simulink model "Statechart_Capsuleuse"  (R2023a)
settings: Solver=FixedStepAuto  StartTime=0.0  StopTime=inf  RelTol=1e-3  EnableMultiTasking=on
libraries: arduinolib x29, simulink x6
settings Model: SimulationMode=external  ExtModeTrigDuration=2  Creator=Renaud  LastModifiedBy=renaud.costadoat
settings SolverCC: AlgebraicLoopSolver=TrustRegion
settings OptimizationCC: EnhancedBackFolding=on  PassReuseOutputArgsAs=Individual arguments  ZeroExternalMemoryAtStartup=off  ZeroInternalMemoryAtStartup=off  MaxStackSize=64  OptimizeBlockOrder=speed  DifferentSizesBufferReuse=on  OptimizationCustomize=off  EfficientTunableParamExpr=on
settings DebuggingCC: ParameterTunabilityLossMsg=error  UnconnectedInputMsg=warning  UnconnectedOutputMsg=warning  UnconnectedLineMsg=warning
settings HardwareCC: ProdBitPerInt=16  ProdBitPerPointer=16  ProdBitPerSizeT=16  ProdBitPerPtrDiffT=16  ProdLargestAtomicFloat=None  ProdWordSize=8  ProdHWDeviceType=Atmel->AVR
settings ModelReferenceCC: EnableRefExpFcnMdlSchedulingChecks=on
settings SFSimCC: MATLABDynamicMemAlloc=off
settings RTWCC: Description=Embedded Coder  SystemTargetFile=ert.tlc  HardwareBoard=Arduino Mega 2560  TemplateMakefile=ert_default_tmf  GenerateReport=on  Toolchain=Arduino AVR  BuildConfiguration=Faster Runs  IncludeHyperlinkInReport=on  LaunchReport=on  GenerateTraceInfo=on  GenerateTraceReport=on  GenerateTraceReportSl=on  GenerateTraceReportSf=on  GenerateTraceReportEml=on
settings CodeAppCC: ForceParamTrailComments=on  IgnoreCustomStorageClasses=off  OperatorAnnotations=on  SimulinkDataObjDesc=on  SFDataObjDesc=on  InsertBlockDesc=on
settings ERTTargetCC: SupportContinuousTime=on  SupportVariableSizeSignals=on  ExtMode=on  ExtModeTransport=3  ExtModeStaticAlloc=on  ExtModeStaticAllocSize=2048  ExtModeMexFile=ext_xcp  ExtModeMexArgs=0 4 921600  ExtModeIntrfLevel=Level2 - Open

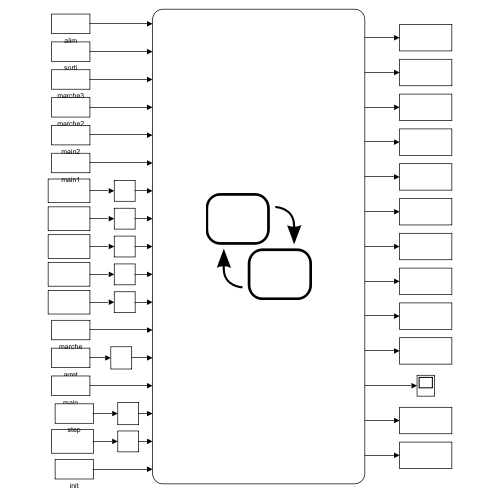
[thumbnail: Simulink's stored preview of the top-level diagram]
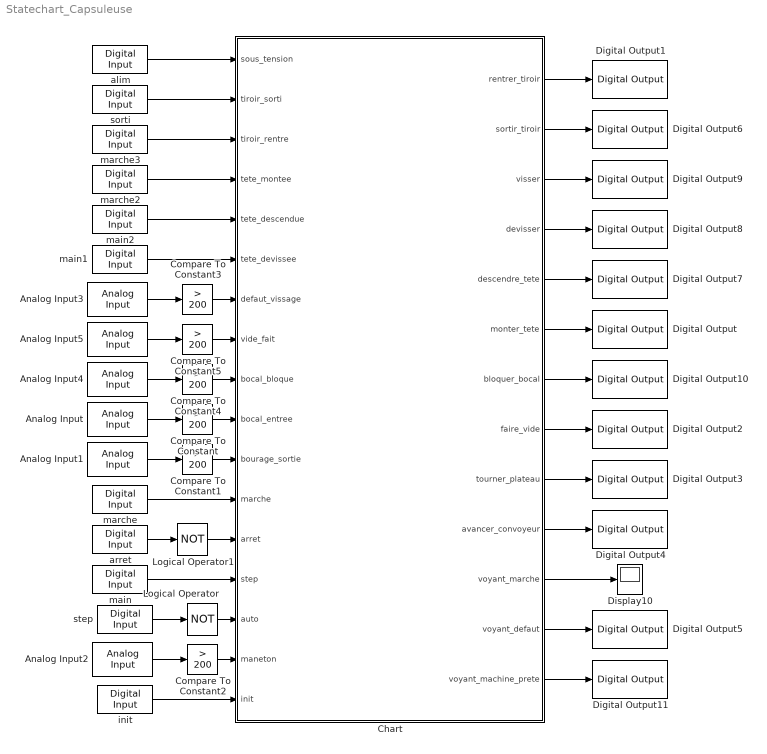
== system Statechart_Capsuleuse ==
  Analog Input : arduinolib/Analog Input  pinNumber=4  ReadResultsOnly=off  ConversionTriggerSource=Software  ExternalTriggerType=uint32( 0 )  OutputDataType=uint16  EnableConversionCompleteNotify=off  EnableOuputStatus=off  SampleTime=-1  blockPlatform=arduino
  Analog Input1 : arduinolib/Analog Input  pinNumber=5  ReadResultsOnly=off  ConversionTriggerSource=Software  ExternalTriggerType=uint32( 0 )  OutputDataType=uint16  EnableConversionCompleteNotify=off  EnableOuputStatus=off  SampleTime=-1  blockPlatform=arduino
  Analog Input2 : arduinolib/Analog Input  pinNumber=3  ReadResultsOnly=off  ConversionTriggerSource=Software  ExternalTriggerType=uint32( 0 )  OutputDataType=uint16  EnableConversionCompleteNotify=off  EnableOuputStatus=off  SampleTime=-1  blockPlatform=arduino
  Analog Input3 : arduinolib/Analog Input  pinNumber=6  ReadResultsOnly=off  ConversionTriggerSource=Software  ExternalTriggerType=uint32( 0 )  OutputDataType=uint16  EnableConversionCompleteNotify=off  EnableOuputStatus=off  SampleTime=-1  blockPlatform=arduino
  Analog Input4 : arduinolib/Analog Input  pinNumber=2  ReadResultsOnly=off  ConversionTriggerSource=Software  ExternalTriggerType=uint32( 0 )  OutputDataType=uint16  EnableConversionCompleteNotify=off  EnableOuputStatus=off  SampleTime=-1  blockPlatform=arduino
  Analog Input5 : arduinolib/Analog Input  pinNumber=1  ReadResultsOnly=off  ConversionTriggerSource=Software  ExternalTriggerType=uint32( 0 )  OutputDataType=uint16  EnableConversionCompleteNotify=off  EnableOuputStatus=off  SampleTime=-1  blockPlatform=arduino
  Chart : Stateflow chart  TreatAsAtomicUnit=on
  Compare To Constant{,1..5} (6 alike) : simulink/Logic and Bit Operations/Compare To Constant  relop=>  const=200  OutDataTypeStr=boolean
  Digital Output : arduinolib/Digital Output  pinNumber=42  Direction=output  blockPlatform=arduino
  Digital Output1 : arduinolib/Digital Output  pinNumber=36  Direction=output  blockPlatform=arduino
  Digital Output10 : arduinolib/Digital Output  pinNumber=5  Direction=output  blockPlatform=arduino
  Digital Output11 : arduinolib/Digital Output  pinNumber=8  Direction=output  blockPlatform=arduino
  Digital Output2 : arduinolib/Digital Output  pinNumber=6  Direction=output  blockPlatform=arduino
  Digital Output3 : arduinolib/Digital Output  pinNumber=43  Direction=output  blockPlatform=arduino
  Digital Output4 : arduinolib/Digital Output  pinNumber=7  Direction=output  blockPlatform=arduino
  Digital Output5 : arduinolib/Digital Output  pinNumber=45  Direction=output  blockPlatform=arduino
  Digital Output6 : arduinolib/Digital Output  pinNumber=37  Direction=output  blockPlatform=arduino
  Digital Output7 : arduinolib/Digital Output  pinNumber=40  Direction=output  blockPlatform=arduino
  Digital Output8 : arduinolib/Digital Output  pinNumber=39  Direction=output  blockPlatform=arduino
  Digital Output9 : arduinolib/Digital Output  pinNumber=38  Direction=output  blockPlatform=arduino
  Display10 : Display
  Logical Operator : Logic  Operator=NOT  AllPortsSameDT=off  OutDataTypeStr=boolean
  Logical Operator1 : Logic  Operator=NOT  AllPortsSameDT=off  OutDataTypeStr=boolean
  alim : arduinolib/Digital Input  pinNumber=22  mode=Default  Direction=input  SampleTime=0.1  blockPlatform=arduino
  arret : arduinolib/Digital Input  pinNumber=31  mode=Default  Direction=input  SampleTime=0.1  blockPlatform=arduino
  init : arduinolib/Digital Input  pinNumber=27  mode=Default  Direction=input  SampleTime=-1  blockPlatform=arduino
  main : arduinolib/Digital Input  pinNumber=29  mode=Default  Direction=input  SampleTime=-1  blockPlatform=arduino
  main1 : arduinolib/Digital Input  pinNumber=3  mode=Default  Direction=input  SampleTime=-1  blockPlatform=arduino
  main2 : arduinolib/Digital Input  pinNumber=2  mode=Default  Direction=input  SampleTime=-1  blockPlatform=arduino
  marche : arduinolib/Digital Input  pinNumber=30  mode=Default  Direction=input  SampleTime=0.1  blockPlatform=arduino
  marche2 : arduinolib/Digital Input  pinNumber=26  mode=Default  Direction=input  SampleTime=0.1  blockPlatform=arduino
  marche3 : arduinolib/Digital Input  pinNumber=25  mode=Default  Direction=input  SampleTime=0.1  blockPlatform=arduino
  sorti : arduinolib/Digital Input  pinNumber=24  mode=Default  Direction=input  SampleTime=-1  blockPlatform=arduino
  step : arduinolib/Digital Input  pinNumber=28  mode=Default  Direction=input  SampleTime=0.1  blockPlatform=arduino
  wires:
  alim/1 -> Chart/1(sous_tension)
  sorti/1 -> Chart/2(tiroir_sorti)
  marche3/1 -> Chart/3(tiroir_rentre)
  marche2/1 -> Chart/4(tete_montee)
  main2/1 -> Chart/5(tete_descendue)
  main1/1 -> Chart/6(tete_devissee)
  Compare To Constant5/1 -> Chart/8(vide_fait)
  Compare To Constant4/1 -> Chart/9(bocal_bloque)
  Compare To Constant/1 -> Chart/10(bocal_entree)
  Compare To Constant1/1 -> Chart/11(bourage_sortie)
  marche/1 -> Chart/12(marche)
  arret/1 -> Logical Operator1/1
  init/1 -> Chart/17(init)
  Chart/1(rentrer_tiroir) -> Digital Output1/1
  Chart/2(sortir_tiroir) -> Digital Output6/1
  Chart/3(visser) -> Digital Output9/1
  Chart/4(devisser) -> Digital Output8/1
  Chart/5(descendre_tete) -> Digital Output7/1
  Chart/6(monter_tete) -> Digital Output/1
  Chart/7(bloquer_bocal) -> Digital Output10/1
  Chart/8(faire_vide) -> Digital Output2/1
  Chart/9(tourner_plateau) -> Digital Output3/1
  Chart/10(avancer_convoyeur) -> Digital Output4/1
  Chart/11(voyant_marche) -> Display10/1
  Chart/12(voyant_defaut) -> Digital Output5/1
  Chart/13(voyant_machine_prete) -> Digital Output11/1
  Compare To Constant2/1 -> Chart/16(maneton)
  main/1 -> Chart/14(step)
  step/1 -> Logical Operator/1
  Analog Input/1 -> Compare To Constant/1
  Analog Input1/1 -> Compare To Constant1/1
  Analog Input2/1 -> Compare To Constant2/1
  Logical Operator/1 -> Chart/15(auto)
  Analog Input3/1 -> Compare To Constant3/1
  Compare To Constant3/1 -> Chart/7(defaut_vissage)
  Analog Input4/1 -> Compare To Constant4/1
  Analog Input5/1 -> Compare To Constant5/1
  Logical Operator1/1 -> Chart/13(arret)

== stateflow chart Statechart_Capsuleuse/Chart ==
  settings: executeAtInitialization=1
  state Fonctionnement
    state Attente_marche
      entry:avancer_convoyeur=0
    state Capsuler
      state Mettre_capsule_sur_bocal [parallel]
        settings: executionOrder=4
        state Init_capsuler
          entry: bocal_pret=0;
          entry: capsule_prete=0;
        state Preparer_bocal_capsule
          state Preparer_capsule [parallel]
            settings: executionOrder=1
            state Sortir_tiroir
              entry:sortir_tiroir=1
              exit:sortir_tiroir=0
            state Descendre_tete
              entry:monter_tete=0
              entry:descendre_tete=1
              exit:descendre_tete=0
            state Faire_vide
              entry:faire_vide=1
            state Monter_tete
              entry:monter_tete=1
              exit:monter_tete=0
            state Rentrer_tiroir
              entry:rentrer_tiroir=1
              exit:rentrer_tiroir=0
            state Capsule_prete
              entry: capsule_prete=1;
            (default) -> Sortir_tiroir
            Sortir_tiroir -> Fonctionnement.Capsuler.Mettre_capsule_sur_bocal.Preparer_bocal_capsule.Preparer_capsule.Descendre_tete : [tiroir_sorti==1]
            Fonctionnement.Capsuler.Mettre_capsule_sur_bocal.Preparer_bocal_capsule.Preparer_capsule.Descendre_tete -> Faire_vide : [tete_descendue==1]
            Faire_vide -> Fonctionnement.Capsuler.Mettre_capsule_sur_bocal.Preparer_bocal_capsule.Preparer_capsule.Monter_tete [order 1] : [vide_fait==1]
            Fonctionnement.Capsuler.Mettre_capsule_sur_bocal.Preparer_bocal_capsule.Preparer_capsule.Monter_tete -> Fonctionnement.Capsuler.Mettre_capsule_sur_bocal.Preparer_bocal_capsule.Preparer_capsule.Rentrer_tiroir : [tete_montee==1]
            Fonctionnement.Capsuler.Mettre_capsule_sur_bocal.Preparer_bocal_capsule.Preparer_capsule.Rentrer_tiroir -> Capsule_prete : [tiroir_rentre==1]
          state Pr_parer_bocal [parallel]
            settings: executionOrder=2
            state Attente_bocal
            state Tourner_plateau
              entry:tourner_plateau=1
              exit:tourner_plateau=0
            state Bloquer_bocal
              entry:bloquer_bocal=1
            state Bocal_pret
              entry: bocal_pret=1;
            (default) -> Attente_bocal
            Attente_bocal -> Fonctionnement.Capsuler.Mettre_capsule_sur_bocal.Preparer_bocal_capsule.Pr_parer_bocal.Tourner_plateau : [bocal_entree==1]
            Fonctionnement.Capsuler.Mettre_capsule_sur_bocal.Preparer_bocal_capsule.Pr_parer_bocal.Tourner_plateau -> Bloquer_bocal : [rising(maneton==1)]
            Bloquer_bocal -> Bocal_pret : [bocal_bloque==1]
        state Descendre_tete
          entry:descendre_tete=1
        state Monter_tete
          entry:descendre_tete=0
          entry:monter_tete=1
          exit:monter_tete=0
        state Devisser
          entry:devisser=1
          exit:devisser=0
        state Visser
          entry:visser=1
          exit:visser=0
          exit:faire_vide=0
        state Faire_vide_liberer_bocal
          entry:bloquer_bocal=0
        (default) -> Init_capsuler
        Fonctionnement.Capsuler.Mettre_capsule_sur_bocal.Devisser -> Init_capsuler [order 1] : [tete_devissee==1 & arret_demande==0]
        Init_capsuler -> Preparer_bocal_capsule : [auto==1|step==1]
        Preparer_bocal_capsule -> Fonctionnement.Capsuler.Mettre_capsule_sur_bocal.Descendre_tete : [capsule_prete==1 & bocal_pret==1]
        Fonctionnement.Capsuler.Mettre_capsule_sur_bocal.Monter_tete -> Fonctionnement.Capsuler.Mettre_capsule_sur_bocal.Devisser : [tete_montee==1]
        Fonctionnement.Capsuler.Mettre_capsule_sur_bocal.Descendre_tete -> Visser : [tete_descendue==1]
        Faire_vide_liberer_bocal -> Fonctionnement.Capsuler.Mettre_capsule_sur_bocal.Monter_tete : [vide_fait==0 && bocal_bloque==0]
        Visser -> Faire_vide_liberer_bocal : [after(1,sec)]
      state Convoyer [parallel]
        settings: executionOrder=3
        state Marche_convoyeur
          entry:avancer_convoyeur=1
        (default) -> Marche_convoyeur
      state Demande_arret [parallel]
        settings: executionOrder=1
        state Attente_arret
          entry:arret_demande=0
        state Arret_demande
          entry:arret_demande=1
        (default) -> Attente_arret
        Attente_arret -> Arret_demande : [arret==1]
      state Voyant_marche [parallel]
        settings: executionOrder=2
        state Allumer_voyant_marche
          entry:voyant_marche=1
          exit:voyant_marche=0
        (default) -> Allumer_voyant_marche
      state Fin_capsules [parallel]
        entry:avancer_convoyeur=0
        settings: executionOrder=5
      Faire_vide -> Fin_capsules [order 2] : [duration(vide_fait==0) > 0.5]
    (default) -> Attente_marche
    Fonctionnement.Capsuler.Mettre_capsule_sur_bocal.Devisser -> Attente_marche [order 2] : [tete_devissee==1 & arret_demande==1]
    Attente_marche -> Capsuler : [marche==1]
  state Attente_mise_en_service
    entry: machine_prete=0;
  state Initialisation
    state Attente_initialisation
      entry:voyant_defaut=0
      entry: PO_en_reference=0;
      entry:faire_vide=0
    state erreur_bourage
      entry:voyant_defaut=1
      exit:voyant_defaut=0
    state Mise_en_PO_reference
      state Monter_tete [parallel]
        entry:monter_tete=1
        settings: executionOrder=1
      state Devisser [parallel]
        entry:devisser=1
        exit:devisser=0
        settings: executionOrder=2
      state Rentrer_tiroir [parallel]
        entry:rentrer_tiroir=1
        exit:rentrer_tiroir=0
        settings: executionOrder=3
      state PO_reference [parallel]
        entry:PO_en_reference=1;
        settings: executionOrder=4
      (default) -> Initialisation.Mise_en_PO_reference.Monter_tete
      Initialisation.Mise_en_PO_reference.Monter_tete -> Initialisation.Mise_en_PO_reference.Devisser : [tete_montee==1]
      Initialisation.Mise_en_PO_reference.Devisser -> Initialisation.Mise_en_PO_reference.Rentrer_tiroir : [tete_devissee==1]
      Initialisation.Mise_en_PO_reference.Rentrer_tiroir -> PO_reference : [tiroir_rentre==1]
    state Tourner_plateau
      entry:tourner_plateau=1
      exit:tourner_plateau=0
    state Machine_prete
      entry:voyant_defaut=0;
      entry:voyant_machine_prete=1
      entry: machine_prete=1
    (default) -> Attente_initialisation
    erreur_bourage -> Attente_initialisation : [bourage_sortie==0]
    (junction 9) -> erreur_bourage [order 1] : [PO_en_reference==1 & bourage_sortie==1]
    Mise_en_PO_reference -> Attente_initialisation [order 2] : [sous_tension==0 ]
    Attente_initialisation -> Mise_en_PO_reference : [init==1 ]
    (junction 9) -> Mise_en_PO_reference [order 3] : [PO_en_reference==0]
    Mise_en_PO_reference -> (junction 9) [order 1] : [PO_en_reference==1]
    (junction 9) -> Initialisation.Tourner_plateau [order 2] : [PO_en_reference==1 & bourage_sortie==0]
    Initialisation.Tourner_plateau -> Machine_prete : [maneton==1]
  (default) -> Attente_mise_en_service
  Fonctionnement -> Attente_mise_en_service : [sous_tension==0 ]
  Initialisation -> Attente_mise_en_service [order 1] : [sous_tension==0 ]
  Attente_mise_en_service -> Initialisation : [sous_tension==1 ]
  Initialisation -> Fonctionnement [order 2] : [machine_prete==1]
  Fin_capsules -> Initialisation
  data: sous_tension input; rentrer_tiroir output =0; sortir_tiroir output; visser output; devisser output =0; descendre_tete output; tiroir_sorti input; tiroir_rentre input; tete_montee input; tete_descendue input; tete_devissee input; defaut_vissage input; vide_fait input; bocal_bloque input; bocal_entree input; bourage_sortie input; marche input; arret input; machine_prete local =0; bocal_pret local =0; capsule_prete local =0; arret_demande local =0; monter_tete output =0; bloquer_bocal output; faire_vide output; tourner_plateau output; avancer_convoyeur output; voyant_marche output; voyant_defaut output; voyant_machine_prete output; PO_en_reference local =0; step input; auto input; maneton input; init input
